simulink model "TST_PTODi_SpdCoord"  (R2016b)
settings: Solver=FixedStepDiscrete  StartTime=0.0  StopTime=simTime  FixedStep=sampleTime  RelTol=1e-3
values from neighbouring files (symbols this model uses):
  testCase = 1    [initTST_PTODi_SpdCoord_001.m]
libraries: simulink x2
settings Model: Creator=Wei Liang  LastModifiedBy=Wei Liang
settings DebuggingCC: SignalRangeChecking=error

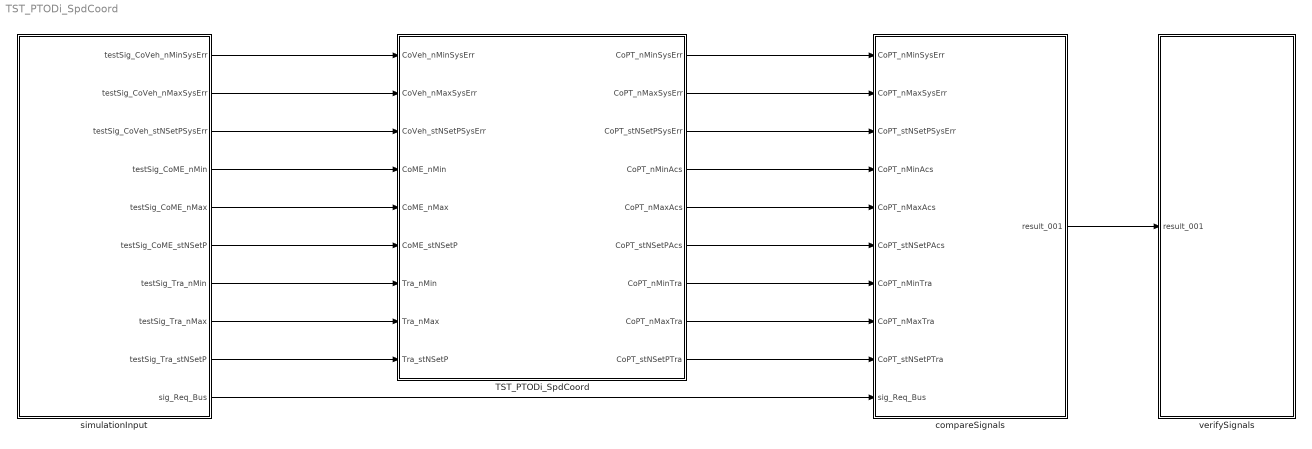
== system TST_PTODi_SpdCoord ==
  TST_PTODi_SpdCoord : Subsystem
  compareSignals : Subsystem
  simulationInput : Subsystem
  verifySignals : Subsystem
  wires:
  simulationInput/1(testSig_CoVeh_nMinSysErr) -> TST_PTODi_SpdCoord/1(CoVeh_nMinSysErr)
  simulationInput/2(testSig_CoVeh_nMaxSysErr) -> TST_PTODi_SpdCoord/2(CoVeh_nMaxSysErr)
  simulationInput/3(testSig_CoVeh_stNSetPSysErr) -> TST_PTODi_SpdCoord/3(CoVeh_stNSetPSysErr)
  simulationInput/4(testSig_CoME_nMin) -> TST_PTODi_SpdCoord/4(CoME_nMin)
  simulationInput/5(testSig_CoME_nMax) -> TST_PTODi_SpdCoord/5(CoME_nMax)
  simulationInput/6(testSig_CoME_stNSetP) -> TST_PTODi_SpdCoord/6(CoME_stNSetP)
  simulationInput/7(testSig_Tra_nMin) -> TST_PTODi_SpdCoord/7(Tra_nMin)
  simulationInput/8(testSig_Tra_nMax) -> TST_PTODi_SpdCoord/8(Tra_nMax)
  simulationInput/9(testSig_Tra_stNSetP) -> TST_PTODi_SpdCoord/9(Tra_stNSetP)
  TST_PTODi_SpdCoord/1(CoPT_nMinSysErr) -> compareSignals/1(CoPT_nMinSysErr)
  TST_PTODi_SpdCoord/2(CoPT_nMaxSysErr) -> compareSignals/2(CoPT_nMaxSysErr)
  TST_PTODi_SpdCoord/3(CoPT_stNSetPSysErr) -> compareSignals/3(CoPT_stNSetPSysErr)
  TST_PTODi_SpdCoord/4(CoPT_nMinAcs) -> compareSignals/4(CoPT_nMinAcs)
  TST_PTODi_SpdCoord/5(CoPT_nMaxAcs) -> compareSignals/5(CoPT_nMaxAcs)
  TST_PTODi_SpdCoord/6(CoPT_stNSetPAcs) -> compareSignals/6(CoPT_stNSetPAcs)
  TST_PTODi_SpdCoord/7(CoPT_nMinTra) -> compareSignals/7(CoPT_nMinTra)
  TST_PTODi_SpdCoord/8(CoPT_nMaxTra) -> compareSignals/8(CoPT_nMaxTra)
  TST_PTODi_SpdCoord/9(CoPT_stNSetPTra) -> compareSignals/9(CoPT_stNSetPTra)
  simulationInput/10(sig_Req_Bus) -> compareSignals/10(sig_Req_Bus)
  compareSignals/1(result_001) -> verifySignals/1(result_001)

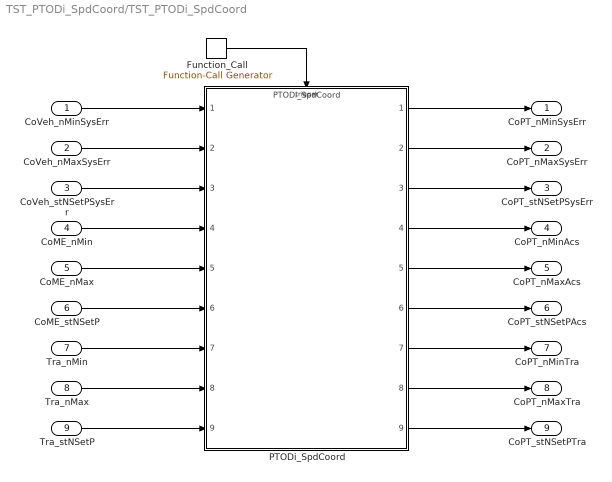
== system TST_PTODi_SpdCoord/TST_PTODi_SpdCoord ==
  CoVeh_nMinSysErr : Inport
  CoVeh_nMaxSysErr : Inport  Port=2
  CoVeh_stNSetPSysErr : Inport  Port=3
  CoME_nMin : Inport  Port=4
  CoME_nMax : Inport  Port=5
  CoME_stNSetP : Inport  Port=6
  Tra_nMin : Inport  Port=7
  Tra_nMax : Inport  Port=8
  Tra_stNSetP : Inport  Port=9
  Function_Call : simulink/Ports & Subsystems/Function-Call Generator  sample_time=sampleTime  numberOfIterations=1
  PTODi_SpdCoord : ModelReference  ModelNameDialog=PTODi_SpdCoord  ModelReferenceVersion=1.3  TriggerPortName=function  TriggerPortTriggerType=function-call  TriggerPortStatesWhenEnabling=held
  CoPT_nMinSysErr : Outport
  CoPT_nMaxSysErr : Outport  Port=2
  CoPT_stNSetPSysErr : Outport  Port=3
  CoPT_nMinAcs : Outport  Port=4
  CoPT_nMaxAcs : Outport  Port=5
  CoPT_stNSetPAcs : Outport  Port=6
  CoPT_nMinTra : Outport  Port=7
  CoPT_nMaxTra : Outport  Port=8
  CoPT_stNSetPTra : Outport  Port=9
  wires:
  Function_Call/1 -> PTODi_SpdCoord/Trigger
  CoVeh_nMinSysErr/1 -> PTODi_SpdCoord/1
  CoVeh_nMaxSysErr/1 -> PTODi_SpdCoord/2
  CoVeh_stNSetPSysErr/1 -> PTODi_SpdCoord/3
  CoME_nMin/1 -> PTODi_SpdCoord/4
  CoME_nMax/1 -> PTODi_SpdCoord/5
  CoME_stNSetP/1 -> PTODi_SpdCoord/6
  Tra_nMin/1 -> PTODi_SpdCoord/7
  Tra_nMax/1 -> PTODi_SpdCoord/8
  Tra_stNSetP/1 -> PTODi_SpdCoord/9
  PTODi_SpdCoord/1 -> CoPT_nMinSysErr/1
  PTODi_SpdCoord/2 -> CoPT_nMaxSysErr/1
  PTODi_SpdCoord/3 -> CoPT_stNSetPSysErr/1
  PTODi_SpdCoord/4 -> CoPT_nMinAcs/1
  PTODi_SpdCoord/5 -> CoPT_nMaxAcs/1
  PTODi_SpdCoord/6 -> CoPT_stNSetPAcs/1
  PTODi_SpdCoord/7 -> CoPT_nMinTra/1
  PTODi_SpdCoord/8 -> CoPT_nMaxTra/1
  PTODi_SpdCoord/9 -> CoPT_stNSetPTra/1

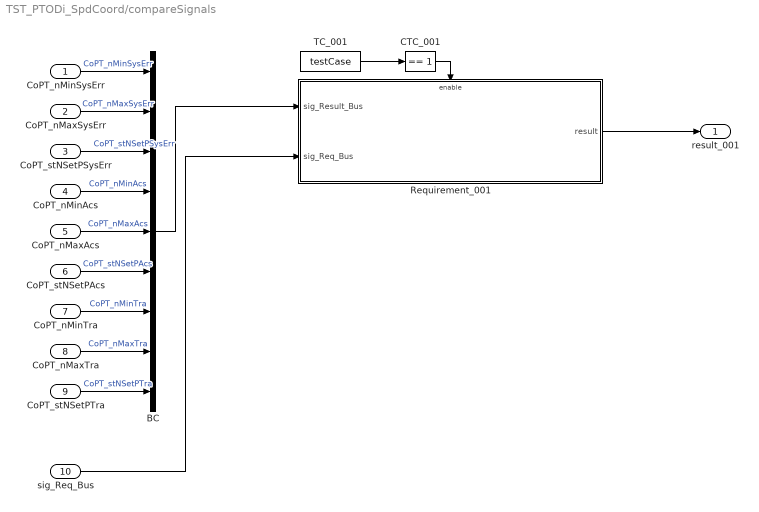
== system TST_PTODi_SpdCoord/compareSignals ==
  CoPT_nMinSysErr : Inport
  CoPT_nMaxSysErr : Inport  Port=2
  CoPT_stNSetPSysErr : Inport  Port=3
  CoPT_nMinAcs : Inport  Port=4
  CoPT_nMaxAcs : Inport  Port=5
  CoPT_stNSetPAcs : Inport  Port=6
  CoPT_nMinTra : Inport  Port=7
  CoPT_nMaxTra : Inport  Port=8
  CoPT_stNSetPTra : Inport  Port=9
  sig_Req_Bus : Inport  Port=10
  BC : BusCreator  Inputs=9
  CTC_001 : simulink/Logic and Bit Operations/Compare To Constant  relop===  const=1  OutDataTypeStr=boolean
  Requirement_001 : Subsystem
  TC_001 : Constant  Value=testCase
  result_001 : Outport
  wires:
  CoPT_nMinSysErr/1 -> BC/1  "CoPT_nMinSysErr"
  CoPT_nMaxSysErr/1 -> BC/2  "CoPT_nMaxSysErr"
  CoPT_stNSetPSysErr/1 -> BC/3  "CoPT_stNSetPSysErr"
  CoPT_nMinAcs/1 -> BC/4  "CoPT_nMinAcs"
  CoPT_nMaxAcs/1 -> BC/5  "CoPT_nMaxAcs"
  CoPT_stNSetPAcs/1 -> BC/6  "CoPT_stNSetPAcs"
  CoPT_nMinTra/1 -> BC/7  "CoPT_nMinTra"
  CoPT_nMaxTra/1 -> BC/8  "CoPT_nMaxTra"
  CoPT_stNSetPTra/1 -> BC/9  "CoPT_stNSetPTra"
  TC_001/1 -> CTC_001/1
  CTC_001/1 -> Requirement_001/Enable
  sig_Req_Bus/1 -> Requirement_001/2(sig_Req_Bus)
  BC/1 -> Requirement_001/1(sig_Result_Bus)
  Requirement_001/1(result) -> result_001/1

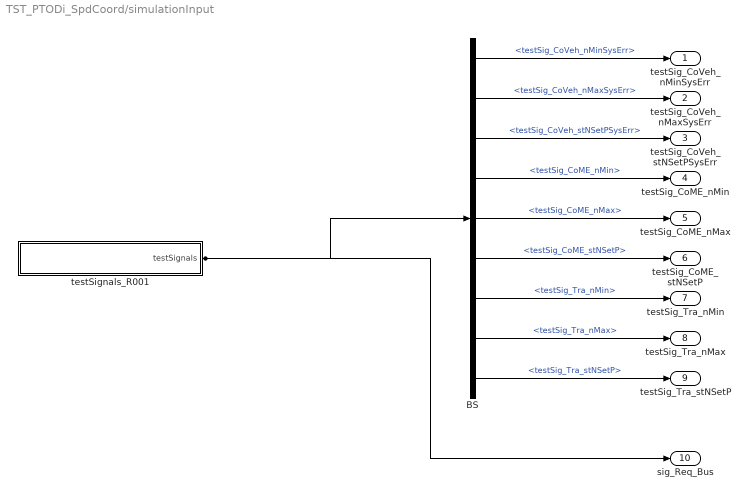
== system TST_PTODi_SpdCoord/simulationInput ==
  BS : BusSelector  OutputSignals=testSig_CoVeh_nMinSysErr,testSig_CoVeh_nMaxSysErr,testSig_CoVeh_stNSetPSysErr,testSig_CoME_nMin,testSig_CoME_nMax,testSig_CoME_stNSetP,testSig_Tra_nMin,testSig_Tra_nMax,testSig_Tra_stNSetP
  testSignals_R001 : Subsystem
  testSig_CoVeh_nMinSysErr : Outport
  testSig_CoVeh_nMaxSysErr : Outport  Port=2
  testSig_CoVeh_stNSetPSysErr : Outport  Port=3
  testSig_CoME_nMin : Outport  Port=4
  testSig_CoME_nMax : Outport  Port=5
  testSig_CoME_stNSetP : Outport  Port=6
  testSig_Tra_nMin : Outport  Port=7
  testSig_Tra_nMax : Outport  Port=8
  testSig_Tra_stNSetP : Outport  Port=9
  sig_Req_Bus : Outport  Port=10
  wires:
  BS/1 -> testSig_CoVeh_nMinSysErr/1  "<testSig_CoVeh_nMinSysErr>"
  BS/2 -> testSig_CoVeh_nMaxSysErr/1  "<testSig_CoVeh_nMaxSysErr>"
  BS/3 -> testSig_CoVeh_stNSetPSysErr/1  "<testSig_CoVeh_stNSetPSysErr>"
  BS/4 -> testSig_CoME_nMin/1  "<testSig_CoME_nMin>"
  BS/5 -> testSig_CoME_nMax/1  "<testSig_CoME_nMax>"
  BS/6 -> testSig_CoME_stNSetP/1  "<testSig_CoME_stNSetP>"
  BS/7 -> testSig_Tra_nMin/1  "<testSig_Tra_nMin>"
  BS/8 -> testSig_Tra_nMax/1  "<testSig_Tra_nMax>"
  BS/9 -> testSig_Tra_stNSetP/1  "<testSig_Tra_stNSetP>"
  testSignals_R001/1(testSignals) -> BS/1, sig_Req_Bus/1

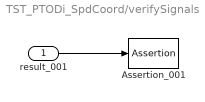
== system TST_PTODi_SpdCoord/verifySignals ==
  result_001 : Inport
  Assertion_001 : Assertion  Enabled=off
  wires:
  result_001/1 -> Assertion_001/1

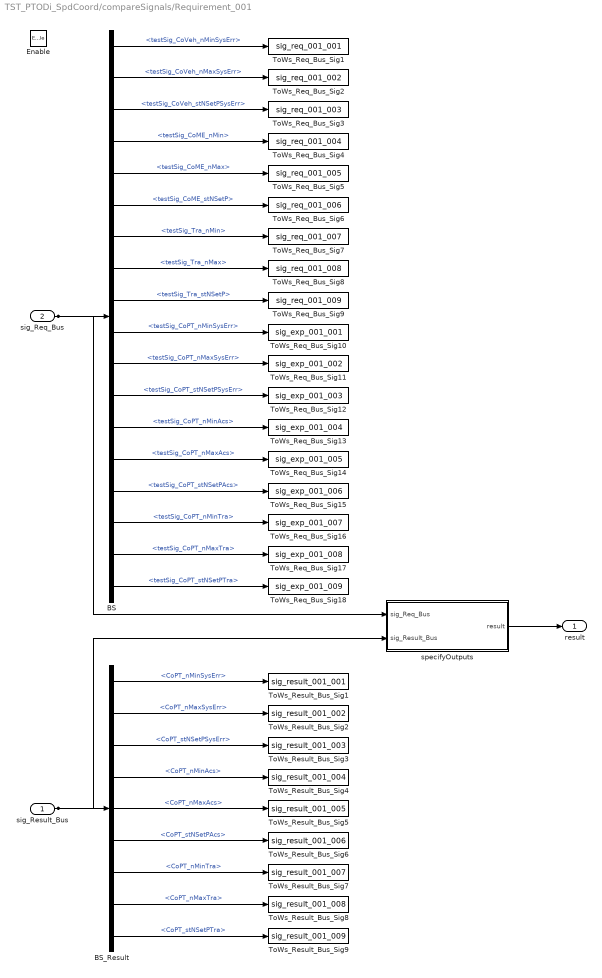
== system TST_PTODi_SpdCoord/compareSignals/Requirement_001 ==
  sig_Result_Bus : Inport
  sig_Req_Bus : Inport  Port=2
  Enable : EnablePort
  BS : BusSelector  OutputSignals=testSig_CoVeh_nMinSysErr,testSig_CoVeh_nMaxSysErr,testSig_CoVeh_stNSetPSysErr,testSig_CoME_nMin,testSig_CoME_nMax,testSig_CoME_stNSetP,testSig_Tra_nMin,testSig_Tra_nMax,testSig_Tra_stNSetP,testSig_CoPT_nMinSysErr,testSig_CoPT_nMaxSysErr,testSig_CoPT_stNSetPSysErr,testSig_CoPT_nMinAcs,testSig_CoPT_nMaxAcs,testSig_CoPT_stNSetPAcs,testSig_CoPT_nMinTra,testSig_CoPT_nMaxTra,testSig_CoPT_stNSetPTra
  BS_Result : BusSelector  OutputSignals=CoPT_nMinSysErr,CoPT_nMaxSysErr,CoPT_stNSetPSysErr,CoPT_nMinAcs,CoPT_nMaxAcs,CoPT_stNSetPAcs,CoPT_nMinTra,CoPT_nMaxTra,CoPT_stNSetPTra
  ToWs_Req_Bus_Sig1 : ToWorkspace  VariableName=sig_req_001_001  SaveFormat=Structure With Time
  ToWs_Req_Bus_Sig10 : ToWorkspace  VariableName=sig_exp_001_001  SaveFormat=Structure With Time
  ToWs_Req_Bus_Sig11 : ToWorkspace  VariableName=sig_exp_001_002  SaveFormat=Structure With Time
  ToWs_Req_Bus_Sig12 : ToWorkspace  VariableName=sig_exp_001_003  SaveFormat=Structure With Time
  ToWs_Req_Bus_Sig13 : ToWorkspace  VariableName=sig_exp_001_004  SaveFormat=Structure With Time
  ToWs_Req_Bus_Sig14 : ToWorkspace  VariableName=sig_exp_001_005  SaveFormat=Structure With Time
  ToWs_Req_Bus_Sig15 : ToWorkspace  VariableName=sig_exp_001_006  SaveFormat=Structure With Time
  ToWs_Req_Bus_Sig16 : ToWorkspace  VariableName=sig_exp_001_007  SaveFormat=Structure With Time
  ToWs_Req_Bus_Sig17 : ToWorkspace  VariableName=sig_exp_001_008  SaveFormat=Structure With Time
  ToWs_Req_Bus_Sig18 : ToWorkspace  VariableName=sig_exp_001_009  SaveFormat=Structure With Time
  ToWs_Req_Bus_Sig2 : ToWorkspace  VariableName=sig_req_001_002  SaveFormat=Structure With Time
  ToWs_Req_Bus_Sig3 : ToWorkspace  VariableName=sig_req_001_003  SaveFormat=Structure With Time
  ToWs_Req_Bus_Sig4 : ToWorkspace  VariableName=sig_req_001_004  SaveFormat=Structure With Time
  ToWs_Req_Bus_Sig5 : ToWorkspace  VariableName=sig_req_001_005  SaveFormat=Structure With Time
  ToWs_Req_Bus_Sig6 : ToWorkspace  VariableName=sig_req_001_006  SaveFormat=Structure With Time
  ToWs_Req_Bus_Sig7 : ToWorkspace  VariableName=sig_req_001_007  SaveFormat=Structure With Time
  ToWs_Req_Bus_Sig8 : ToWorkspace  VariableName=sig_req_001_008  SaveFormat=Structure With Time
  ToWs_Req_Bus_Sig9 : ToWorkspace  VariableName=sig_req_001_009  SaveFormat=Structure With Time
  ToWs_Result_Bus_Sig1 : ToWorkspace  VariableName=sig_result_001_001  SaveFormat=Structure With Time
  ToWs_Result_Bus_Sig2 : ToWorkspace  VariableName=sig_result_001_002  SaveFormat=Structure With Time
  ToWs_Result_Bus_Sig3 : ToWorkspace  VariableName=sig_result_001_003  SaveFormat=Structure With Time
  ToWs_Result_Bus_Sig4 : ToWorkspace  VariableName=sig_result_001_004  SaveFormat=Structure With Time
  ToWs_Result_Bus_Sig5 : ToWorkspace  VariableName=sig_result_001_005  SaveFormat=Structure With Time
  ToWs_Result_Bus_Sig6 : ToWorkspace  VariableName=sig_result_001_006  SaveFormat=Structure With Time
  ToWs_Result_Bus_Sig7 : ToWorkspace  VariableName=sig_result_001_007  SaveFormat=Structure With Time
  ToWs_Result_Bus_Sig8 : ToWorkspace  VariableName=sig_result_001_008  SaveFormat=Structure With Time
  ToWs_Result_Bus_Sig9 : ToWorkspace  VariableName=sig_result_001_009  SaveFormat=Structure With Time
  specifyOutputs : Subsystem
  result : Outport
  wires:
  sig_Req_Bus/1 -> BS/1, specifyOutputs/1(sig_Req_Bus)
  BS/1 -> ToWs_Req_Bus_Sig1/1  "<testSig_CoVeh_nMinSysErr>"
  BS/2 -> ToWs_Req_Bus_Sig2/1  "<testSig_CoVeh_nMaxSysErr>"
  BS/3 -> ToWs_Req_Bus_Sig3/1  "<testSig_CoVeh_stNSetPSysErr>"
  BS/4 -> ToWs_Req_Bus_Sig4/1  "<testSig_CoME_nMin>"
  BS/5 -> ToWs_Req_Bus_Sig5/1  "<testSig_CoME_nMax>"
  BS/6 -> ToWs_Req_Bus_Sig6/1  "<testSig_CoME_stNSetP>"
  BS/7 -> ToWs_Req_Bus_Sig7/1  "<testSig_Tra_nMin>"
  BS/8 -> ToWs_Req_Bus_Sig8/1  "<testSig_Tra_nMax>"
  BS/9 -> ToWs_Req_Bus_Sig9/1  "<testSig_Tra_stNSetP>"
  BS/10 -> ToWs_Req_Bus_Sig10/1  "<testSig_CoPT_nMinSysErr>"
  BS/11 -> ToWs_Req_Bus_Sig11/1  "<testSig_CoPT_nMaxSysErr>"
  BS/12 -> ToWs_Req_Bus_Sig12/1  "<testSig_CoPT_stNSetPSysErr>"
  BS/13 -> ToWs_Req_Bus_Sig13/1  "<testSig_CoPT_nMinAcs>"
  BS/14 -> ToWs_Req_Bus_Sig14/1  "<testSig_CoPT_nMaxAcs>"
  BS/15 -> ToWs_Req_Bus_Sig15/1  "<testSig_CoPT_stNSetPAcs>"
  BS/16 -> ToWs_Req_Bus_Sig16/1  "<testSig_CoPT_nMinTra>"
  BS/17 -> ToWs_Req_Bus_Sig17/1  "<testSig_CoPT_nMaxTra>"
  BS/18 -> ToWs_Req_Bus_Sig18/1  "<testSig_CoPT_stNSetPTra>"
  sig_Result_Bus/1 -> BS_Result/1, specifyOutputs/2(sig_Result_Bus)
  BS_Result/1 -> ToWs_Result_Bus_Sig1/1  "<CoPT_nMinSysErr>"
  BS_Result/2 -> ToWs_Result_Bus_Sig2/1  "<CoPT_nMaxSysErr>"
  BS_Result/3 -> ToWs_Result_Bus_Sig3/1  "<CoPT_stNSetPSysErr>"
  BS_Result/4 -> ToWs_Result_Bus_Sig4/1  "<CoPT_nMinAcs>"
  BS_Result/5 -> ToWs_Result_Bus_Sig5/1  "<CoPT_nMaxAcs>"
  BS_Result/6 -> ToWs_Result_Bus_Sig6/1  "<CoPT_stNSetPAcs>"
  BS_Result/7 -> ToWs_Result_Bus_Sig7/1  "<CoPT_nMinTra>"
  BS_Result/8 -> ToWs_Result_Bus_Sig8/1  "<CoPT_nMaxTra>"
  BS_Result/9 -> ToWs_Result_Bus_Sig9/1  "<CoPT_stNSetPTra>"
  specifyOutputs/1(result) -> result/1

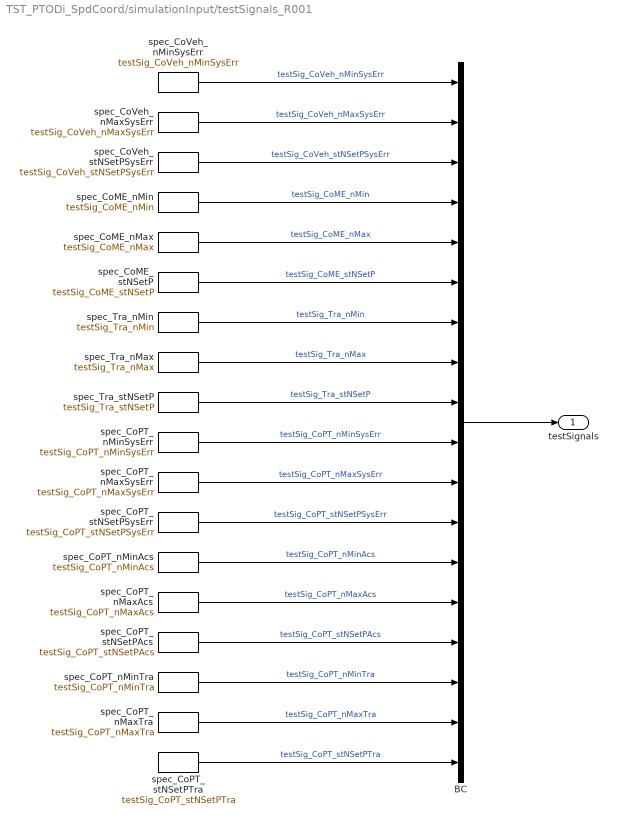
== system TST_PTODi_SpdCoord/simulationInput/testSignals_R001 ==
  BC : BusCreator  Inputs=18
  spec_CoME_nMax : FromWorkspace  VariableName=testSig_CoME_nMax  Interpolate=off  OutputAfterFinalValue=Holding final value
  spec_CoME_nMin : FromWorkspace  VariableName=testSig_CoME_nMin  Interpolate=off  OutputAfterFinalValue=Holding final value
  spec_CoME_stNSetP : FromWorkspace  VariableName=testSig_CoME_stNSetP  Interpolate=off  OutputAfterFinalValue=Holding final value
  spec_CoPT_nMaxAcs : FromWorkspace  VariableName=testSig_CoPT_nMaxAcs  Interpolate=off  OutputAfterFinalValue=Holding final value
  spec_CoPT_nMaxSysErr : FromWorkspace  VariableName=testSig_CoPT_nMaxSysErr  Interpolate=off  OutputAfterFinalValue=Holding final value
  spec_CoPT_nMaxTra : FromWorkspace  VariableName=testSig_CoPT_nMaxTra  Interpolate=off  OutputAfterFinalValue=Holding final value
  spec_CoPT_nMinAcs : FromWorkspace  VariableName=testSig_CoPT_nMinAcs  Interpolate=off  OutputAfterFinalValue=Holding final value
  spec_CoPT_nMinSysErr : FromWorkspace  VariableName=testSig_CoPT_nMinSysErr  Interpolate=off  OutputAfterFinalValue=Holding final value
  spec_CoPT_nMinTra : FromWorkspace  VariableName=testSig_CoPT_nMinTra  Interpolate=off  OutputAfterFinalValue=Holding final value
  spec_CoPT_stNSetPAcs : FromWorkspace  VariableName=testSig_CoPT_stNSetPAcs  Interpolate=off  OutputAfterFinalValue=Holding final value
  spec_CoPT_stNSetPSysErr : FromWorkspace  VariableName=testSig_CoPT_stNSetPSysErr  Interpolate=off  OutputAfterFinalValue=Holding final value
  spec_CoPT_stNSetPTra : FromWorkspace  VariableName=testSig_CoPT_stNSetPTra  Interpolate=off  OutputAfterFinalValue=Holding final value
  spec_CoVeh_nMaxSysErr : FromWorkspace  VariableName=testSig_CoVeh_nMaxSysErr  Interpolate=off  OutputAfterFinalValue=Holding final value
  spec_CoVeh_nMinSysErr : FromWorkspace  VariableName=testSig_CoVeh_nMinSysErr  Interpolate=off  OutputAfterFinalValue=Holding final value
  spec_CoVeh_stNSetPSysErr : FromWorkspace  VariableName=testSig_CoVeh_stNSetPSysErr  Interpolate=off  OutputAfterFinalValue=Holding final value
  spec_Tra_nMax : FromWorkspace  VariableName=testSig_Tra_nMax  Interpolate=off  OutputAfterFinalValue=Holding final value
  spec_Tra_nMin : FromWorkspace  VariableName=testSig_Tra_nMin  Interpolate=off  OutputAfterFinalValue=Holding final value
  spec_Tra_stNSetP : FromWorkspace  VariableName=testSig_Tra_stNSetP  Interpolate=off  OutputAfterFinalValue=Holding final value
  testSignals : Outport
  wires:
  BC/1 -> testSignals/1
  spec_CoVeh_nMinSysErr/1 -> BC/1  "testSig_CoVeh_nMinSysErr"
  spec_CoVeh_nMaxSysErr/1 -> BC/2  "testSig_CoVeh_nMaxSysErr"
  spec_CoVeh_stNSetPSysErr/1 -> BC/3  "testSig_CoVeh_stNSetPSysErr"
  spec_CoME_nMin/1 -> BC/4  "testSig_CoME_nMin"
  spec_CoME_nMax/1 -> BC/5  "testSig_CoME_nMax"
  spec_CoME_stNSetP/1 -> BC/6  "testSig_CoME_stNSetP"
  spec_Tra_nMin/1 -> BC/7  "testSig_Tra_nMin"
  spec_Tra_nMax/1 -> BC/8  "testSig_Tra_nMax"
  spec_Tra_stNSetP/1 -> BC/9  "testSig_Tra_stNSetP"
  spec_CoPT_nMinSysErr/1 -> BC/10  "testSig_CoPT_nMinSysErr"
  spec_CoPT_nMaxSysErr/1 -> BC/11  "testSig_CoPT_nMaxSysErr"
  spec_CoPT_stNSetPSysErr/1 -> BC/12  "testSig_CoPT_stNSetPSysErr"
  spec_CoPT_nMinAcs/1 -> BC/13  "testSig_CoPT_nMinAcs"
  spec_CoPT_nMaxAcs/1 -> BC/14  "testSig_CoPT_nMaxAcs"
  spec_CoPT_stNSetPAcs/1 -> BC/15  "testSig_CoPT_stNSetPAcs"
  spec_CoPT_nMinTra/1 -> BC/16  "testSig_CoPT_nMinTra"
  spec_CoPT_nMaxTra/1 -> BC/17  "testSig_CoPT_nMaxTra"
  spec_CoPT_stNSetPTra/1 -> BC/18  "testSig_CoPT_stNSetPTra"

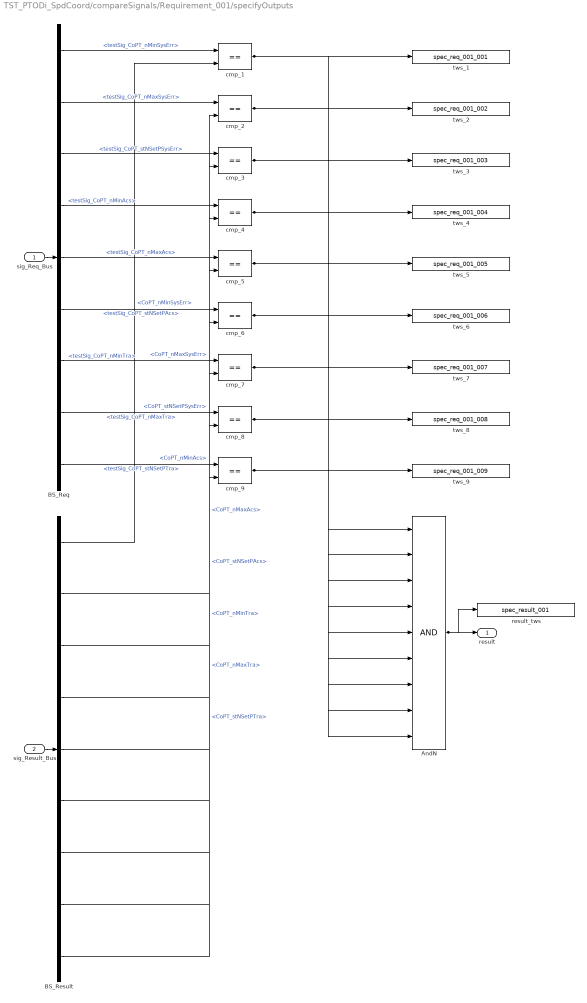
== system TST_PTODi_SpdCoord/compareSignals/Requirement_001/specifyOutputs ==
  sig_Req_Bus : Inport
  sig_Result_Bus : Inport  Port=2
  AndN : Logic  Inputs=9
  BS_Req : BusSelector  OutputSignals=testSig_CoPT_nMinSysErr,testSig_CoPT_nMaxSysErr,testSig_CoPT_stNSetPSysErr,testSig_CoPT_nMinAcs,testSig_CoPT_nMaxAcs,testSig_CoPT_stNSetPAcs,testSig_CoPT_nMinTra,testSig_CoPT_nMaxTra,testSig_CoPT_stNSetPTra
  BS_Result : BusSelector  OutputSignals=CoPT_nMinSysErr,CoPT_nMaxSysErr,CoPT_stNSetPSysErr,CoPT_nMinAcs,CoPT_nMaxAcs,CoPT_stNSetPAcs,CoPT_nMinTra,CoPT_nMaxTra,CoPT_stNSetPTra
  cmp_{1..9} (9 alike) : RelationalOperator  Operator===  RndMeth=Nearest  InputSameDT=on
  result_tws : ToWorkspace  VariableName=spec_result_001
  tws_1 : ToWorkspace  VariableName=spec_req_001_001
  tws_2 : ToWorkspace  VariableName=spec_req_001_002
  tws_3 : ToWorkspace  VariableName=spec_req_001_003
  tws_4 : ToWorkspace  VariableName=spec_req_001_004
  tws_5 : ToWorkspace  VariableName=spec_req_001_005
  tws_6 : ToWorkspace  VariableName=spec_req_001_006
  tws_7 : ToWorkspace  VariableName=spec_req_001_007
  tws_8 : ToWorkspace  VariableName=spec_req_001_008
  tws_9 : ToWorkspace  VariableName=spec_req_001_009
  result : Outport
  wires:
  sig_Req_Bus/1 -> BS_Req/1
  sig_Result_Bus/1 -> BS_Result/1
  AndN/1 -> result/1, result_tws/1
  BS_Req/1 -> cmp_1/1  "<testSig_CoPT_nMinSysErr>"
  BS_Result/1 -> cmp_1/2  "<CoPT_nMinSysErr>"
  cmp_1/1 -> tws_1/1, AndN/1
  BS_Req/2 -> cmp_2/1  "<testSig_CoPT_nMaxSysErr>"
  BS_Result/2 -> cmp_2/2  "<CoPT_nMaxSysErr>"
  cmp_2/1 -> tws_2/1, AndN/2
  BS_Req/3 -> cmp_3/1  "<testSig_CoPT_stNSetPSysErr>"
  BS_Result/3 -> cmp_3/2  "<CoPT_stNSetPSysErr>"
  cmp_3/1 -> tws_3/1, AndN/3
  BS_Req/4 -> cmp_4/1  "<testSig_CoPT_nMinAcs>"
  BS_Result/4 -> cmp_4/2  "<CoPT_nMinAcs>"
  cmp_4/1 -> tws_4/1, AndN/4
  BS_Req/5 -> cmp_5/1  "<testSig_CoPT_nMaxAcs>"
  BS_Result/5 -> cmp_5/2  "<CoPT_nMaxAcs>"
  cmp_5/1 -> tws_5/1, AndN/5
  BS_Req/6 -> cmp_6/1  "<testSig_CoPT_stNSetPAcs>"
  BS_Result/6 -> cmp_6/2  "<CoPT_stNSetPAcs>"
  cmp_6/1 -> tws_6/1, AndN/6
  BS_Req/7 -> cmp_7/1  "<testSig_CoPT_nMinTra>"
  BS_Result/7 -> cmp_7/2  "<CoPT_nMinTra>"
  cmp_7/1 -> tws_7/1, AndN/7
  BS_Req/8 -> cmp_8/1  "<testSig_CoPT_nMaxTra>"
  BS_Result/8 -> cmp_8/2  "<CoPT_nMaxTra>"
  cmp_8/1 -> tws_8/1, AndN/8
  BS_Req/9 -> cmp_9/1  "<testSig_CoPT_stNSetPTra>"
  BS_Result/9 -> cmp_9/2  "<CoPT_stNSetPTra>"
  cmp_9/1 -> tws_9/1, AndN/9
